simulink model "pitch_rate_command"  (R2018a)
settings: Solver=VariableStepAuto  StartTime=0.0  StopTime=100  RelTol=1e-3
values from neighbouring files (symbols this model uses):
  trim_control_lin = trim_control_lo    [FindF16Dynamics.m]    (also in FindF16DynamicsCanyon.m; chap5data.mat = [-2.46068617229 3.21143579128e-16 2.79661206579e-15]; data.mat = [-2.46068617229 3.21143579128e-16 2.79661206579e-15])
settings Model: Creator=maesj  LastModifiedBy=maesj

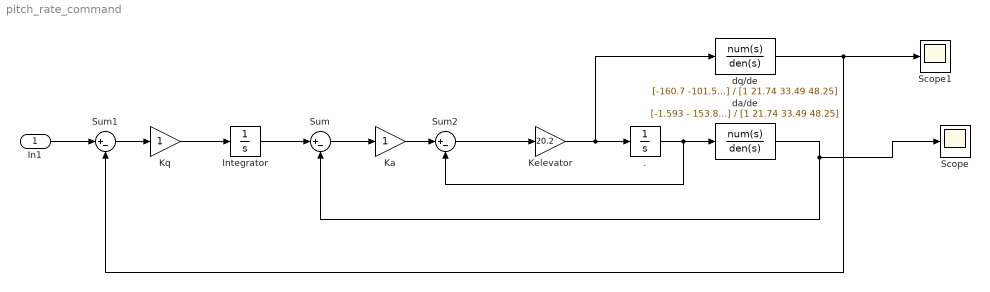
== system pitch_rate_command ==
  In1 : Inport
  . : Integrator  InitialCondition=trim_control_lin(1)
  Integrator : Integrator
  Ka : Gain
  Kelevator : Gain  Gain=20.2
  Kq : Gain
  Scope : Scope
  Scope1 : Scope
  Sum : Sum  Inputs=|+-
  Sum1 : Sum  Inputs=|+-
  Sum2 : Sum  Inputs=|+-
  da/de : TransferFcn  Numerator=[-1.593 - 153.8]  Denominator=[1 21.74 33.49 48.25]
  dq/de : TransferFcn  Numerator=[-160.7 -101.5]  Denominator=[1 21.74 33.49 48.25]
  wires:
  Kq/1 -> Integrator/1
  da/de/1 -> Scope/1, Sum/2
  Integrator/1 -> Sum/1
  Sum1/1 -> Kq/1
  Sum/1 -> Ka/1
  Sum2/1 -> Kelevator/1
  Kelevator/1 -> dq/de/1, ./1
  Ka/1 -> Sum2/1
  ./1 -> da/de/1, Sum2/2
  In1/1 -> Sum1/1
  dq/de/1 -> Scope1/1, Sum1/2
